simulink model "pioneer_stop_obstacle"  (R2022b)
settings: Solver=ode3  StartTime=0.0  StopTime=inf  FixedStep=0.02  RelTol=1e-3
model workspace (MAT data in the model file):
  Logfile_Data_Object : robotics.ros.BagSelection (value not decoded)
  Logfile_Path = 'C:\Users\user\Desktop\camera2022-04-27-13-31-43.bag'
  Logfile_Playback_Duration = nan
  Logfile_Playback_Offset = nan
undefined symbols (not defined in the file): Angular, Linear, waypoints211
libraries: robotlib x5, robotcorelib x1, robotalgslib x1
settings Model: SimulationMode=external  Creator=user  LastModifiedBy=tarun
settings SolverCC: AlgebraicLoopSolver=TrustRegion
settings OptimizationCC: EnhancedBackFolding=on  PassReuseOutputArgsAs=Individual arguments  ZeroExternalMemoryAtStartup=off  ZeroInternalMemoryAtStartup=off  MaxStackSize=64  OptimizeBlockOrder=speed  DifferentSizesBufferReuse=on  OptimizationCustomize=off  EfficientTunableParamExpr=on
settings DebuggingCC: ParameterTunabilityLossMsg=error  UnconnectedInputMsg=warning  UnconnectedOutputMsg=warning  UnconnectedLineMsg=warning  SFMachineParentedDataDiag=warning
settings HardwareCC: ProdBitPerPointer=32  ProdBitPerSizeT=32  ProdBitPerPtrDiffT=32  ProdLargestAtomicFloat=None  ProdIntDivRoundTo=Undefined  ProdEndianess=Unspecified  ProdWordSize=32  ProdHWDeviceType=Generic->Unspecified (assume 32-bit Generic)
settings ModelReferenceCC: EnableRefExpFcnMdlSchedulingChecks=on
settings SFSimCC: MATLABDynamicMemAlloc=off  SimTargetLang=C++
settings RTWCC: Description=Embedded Coder  SystemTargetFile=ert.tlc  HardwareBoard=Robot Operating System (ROS)  TLCOptions="-aInlineSetEventsForThisBaseRateFcn=TLC_FALSE -aSuppressMultiTaskScheduler=TLC_FALSE  -aRateBasedStepFcn=0"  TemplateMakefile=ert_default_tmf  Toolchain=Catkin  TargetLang=C++  DLArmComputeVersion=19.05
settings CodeAppCC: ForceParamTrailComments=on  IgnoreCustomStorageClasses=off  OperatorAnnotations=on  SimulinkDataObjDesc=on  SFDataObjDesc=on  InsertBlockDesc=on
settings ERTTargetCC: ExtMode=on  ExtModeMexArgs='192.168.232.176' 0 17725

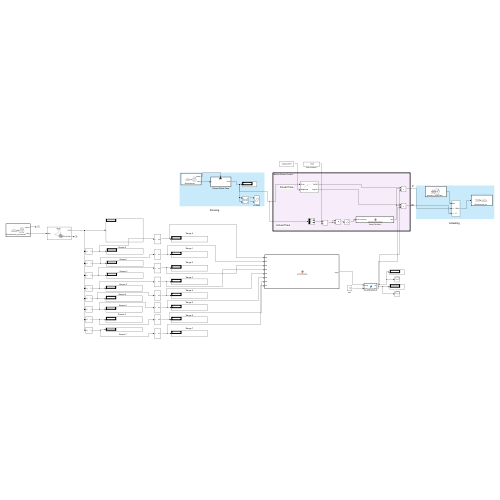
[thumbnail: Simulink's stored preview of the top-level diagram]
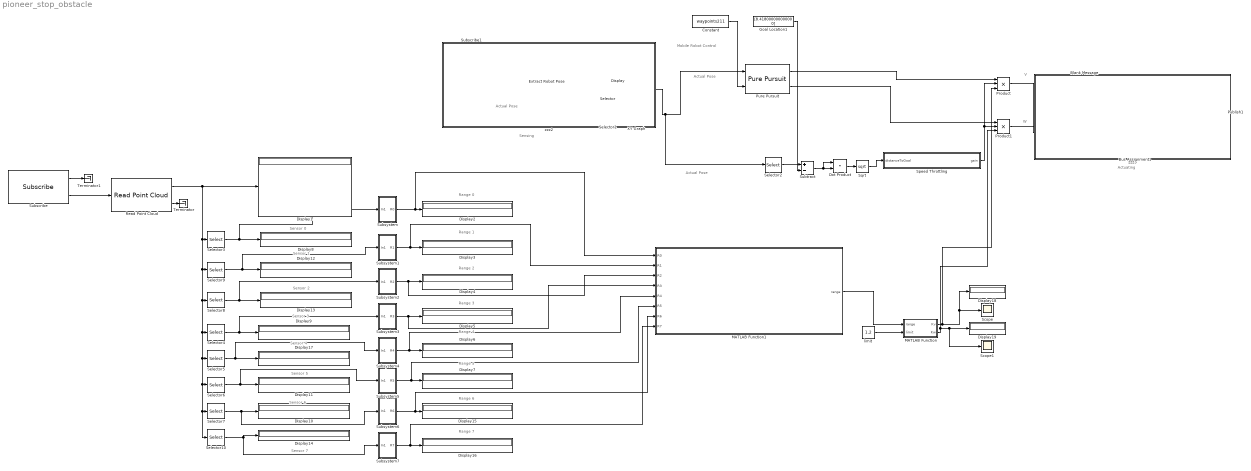
== system pioneer_stop_obstacle ==
  note: Sensing
  note: Sensor 2
  note: Range 6
  note: Actual Pose
  note: Actual Pose
  note: V
  note: Sensor 3
  note: Sensor 4
  note: Mobile Robot Control
  note: Sensor 5
  note: Sensor 0
  note: Range 3
  note: Range 0
  note: Sensor 1
  note: Range 5
  note: Range 7
  note: W
  note: Range 1
  note: Sensor 6
  note: Sensor 7
  note: Range 2
  note: Actual Pose
  note: Range 4
  note: Actuating
  Blank Message : robotlib/Blank Message  messageClass=Message  entityType=geometry_msgs/Twist  messageType=geometry_msgs/Twist  SampleTime=inf  legacyBusStruct=off
  Bus Assignment1 : BusAssignment  AssignedSignals=Linear.X,Angular.Z
  Constant : Constant  Value=waypoints211
  Display{,1..19} (20 alike) : Display
  Dot Product : DotProduct  OutDataTypeStr=Inherit: Inherit via internal rule
  Extract Robot Pose : Subsystem
  Goal Location1 : Constant  Value="[8.41800000000000\t0]"
  MATLAB Function : MATLAB Function  TreatAsAtomicUnit=on
  MATLAB Function1 : MATLAB Function  TreatAsAtomicUnit=on
  Product : Product  Inputs=3
  Product1 : Product  Inputs=3
  Publish1 : robotlib/Publish  topicSource=Select from ROS network  topic=/RosAria/cmd_vel  messageType=geometry_msgs/Twist  legacyBusStruct=off  messageQueueLength=105
  Pure Pursuit : robotalgslib/Pure Pursuit  DesiredLinearVelocity=0.3  MaxAngularVelocity=0.8  LookaheadDistance=1  TargetDirPort=off  SimulateUsing=Code generation
  Read Point Cloud : robotlib/Read Point Cloud  MaximumPointCloudSize=[8, 1]  PreserveStructure=off  ShowRGBOutput=off  ShowIntensityOutput=off  ShowErrorCodeOutput=on  VariableSizeOutputs=off
  Scope : Scope
  Scope1 : Scope
  Selector : Selector  InputPortWidth=3  IndexOptions=Index vector (dialog)  Indices=[1]  OutputSizes=1
  Selector1 : Selector  InputPortWidth=3  IndexOptions=Index vector (dialog)  Indices=[2]  OutputSizes=1
  Selector10 : Selector  NumberOfDimensions=2  InputPortWidth=6  IndexOptions=Starting index (dialog),Starting index (dialog)  Indices=8,1  OutputSizes=1,3
  Selector2 : Selector  InputPortWidth=3  IndexOptions=Index vector (dialog)  Indices=[1 2]  OutputSizes=1
  Selector3 : Selector  NumberOfDimensions=2  InputPortWidth=6  IndexOptions=Starting index (dialog),Starting index (dialog)  Indices=1,1  OutputSizes=1,3
  Selector4 : Selector  NumberOfDimensions=2  InputPortWidth=6  IndexOptions=Starting index (dialog),Starting index (dialog)  Indices=4,1  OutputSizes=1,3
  Selector5 : Selector  NumberOfDimensions=2  InputPortWidth=6  IndexOptions=Starting index (dialog),Starting index (dialog)  Indices=5,1  OutputSizes=1,3
  Selector6 : Selector  NumberOfDimensions=2  InputPortWidth=6  IndexOptions=Starting index (dialog),Starting index (dialog)  Indices=6,1  OutputSizes=1,3
  Selector7 : Selector  NumberOfDimensions=2  InputPortWidth=6  IndexOptions=Starting index (dialog),Starting index (dialog)  Indices=7,1  OutputSizes=1,3
  Selector8 : Selector  NumberOfDimensions=2  InputPortWidth=6  IndexOptions=Starting index (dialog),Starting index (dialog)  Indices=3,1  OutputSizes=1,3
  Selector9 : Selector  NumberOfDimensions=2  InputPortWidth=6  IndexOptions=Starting index (dialog),Starting index (dialog)  Indices=2,1  OutputSizes=1,3
  Speed Throttling : MATLAB Function  TreatAsAtomicUnit=on
  Sqrt : Sqrt
  Subscribe : robotlib/Subscribe  topicSource=Select from ROS network  topic=/RosAria/sonar_pointcloud2  messageType=sensor_msgs/PointCloud2  SampleTime=0.02  legacyBusStruct=off  messageQueueLength=1
  Subscribe1 : robotlib/Subscribe  topicSource=Select from ROS network  topic=/RosAria/pose  messageType=nav_msgs/Odometry  SampleTime=0.02  legacyBusStruct=off  messageQueueLength=51
  Subsystem : Subsystem
  Subsystem1 : Subsystem
  Subsystem2 : Subsystem
  Subsystem3 : Subsystem
  Subsystem4 : Subsystem
  Subsystem5 : Subsystem
  Subsystem6 : Subsystem
  Subsystem7 : Subsystem
  Subtract : Sum  Inputs=+-
  Terminator : Terminator
  Terminator1 : Terminator
  XY Graph : Record  FileSettingsInternal="{\"entries\":[{\"content\":{\"excelSettings\":{\"content\":{},\"type\":\"Streamout.ExcelSettings\"}},\"type\":\"Streamout.FileSettingStorage\",\"uuid\":\"6dcafb8c-c2e8-42d2-a393-42a68d2ab7a7\"}],\"packageUris\":[\"http://schema.mathworks.com/mf0/streamout_blocks/R2020a\"],\"version\":\"1.0\"}"  Layout=[1 1]  SignalsInternal="{\"entries\":[{\"content\":{\"signals\":[{\"content\":{\"blockPath\":[\"pioneer_stop_obstacle/XY Graph\"],\"channel\":[],\"dimensions\":[1],\"domain\":\"pioneer_stop_obstacle/XY Graph\",\"lineColor\":\"#a2142f\",\"plots\":[1],\"port\":1,\"sid\":[],\"signalID\":34,\"signalName\":\"XY Graph:1\"},\"type\":\"RecordBlkView.Signal\",\"uuid\":\"3db1dab7-281e-4972-95fd-2f43a7dd423c\"},{\"content\":{\"blockPath\":[\"pioneer_stop_obstacle/XY Graph\"],\"channel\":[],\"dimensions\":[1],\"domain\":\"pioneer_stop_obstacle/XY Graph\",\"lineColor\":\"#139fff\",\"plots\":[1],\"port\":2,\"sid\":[],\"signalID\":37,\"signalName\":\"XY Graph:2\"},\"type\":\"RecordBlkView.Signal\",\"uuid\":\"8cbd3084-6a6a-4caa-acfe-6605f40577f9\"}]},\"type\":\"RecordBlkView.InputSignals\",\"uuid\":\"3c1224c5-a623-4e21-a2bc-4ee778cdb473\"}],\"packageUris\":[\"http://schema.mathworks.com/mf0/streamout_blocks/R2020a\"],\"version\":\"1.0\"}"  VisualizationBindings="{\"xyplotplugin\":{\"info\":[{\"series\":[{\"bindingParametersList\":[{\"parameter\":\"X-Axis\",\"signalID\":34,\"signalName\":\"XY Graph:1\"},{\"parameter\":\"Y-Axis\",\"signalID\":37,\"signalName\":\"XY Graph:2\"}],\"seriesID\":47604}],\"subplotID\":1}]}}"  CompatibilityTag=XY  st=-1
  limit : Constant  Value=1.2
  zzz2 : Subsystem  TreatAsAtomicUnit=on
      settings: OpenFcn=% no-op
      mask Display: disp('')
  zzz3 : Subsystem  TreatAsAtomicUnit=on
      settings: OpenFcn=% no-op
      mask Display: disp('')
  wires:
  Selector9/1 -> Subsystem1/1(In1), Display12/1
  Subsystem5/1(R5) -> MATLAB Function1/6(R5), Display7/1
  Selector5/1 -> Subsystem4/1(In1), Display17/1
  Selector10/1 -> Subsystem7/1(In1), Display14/1
  Subsystem3/1(R3) -> MATLAB Function1/4(R3), Display5/1
  Selector7/1 -> Subsystem6/1(In1), Display10/1
  Blank Message/1 -> Bus Assignment1/1
  Selector6/1 -> Subsystem5/1(In1), Display11/1
  Subscribe/2 -> Read Point Cloud/1
  Selector/1 -> XY Graph/1
  Read Point Cloud/1 -> Selector10/1, Selector7/1, Selector6/1, Selector5/1, Selector4/1, Selector8/1, Selector9/1, Selector3/1, Display1/1
  Constant/1 -> Pure Pursuit/2
  Product1/1 -> Bus Assignment1/3
  Subsystem7/1(R7) -> MATLAB Function1/8(R7), Display16/1
  Selector3/1 -> Subsystem/1(In1), Display8/1
  Selector4/1 -> Subsystem3/1(In1), Display9/1
  Subsystem6/1(R6) -> MATLAB Function1/7(R6), Display15/1
  Selector1/1 -> XY Graph/2
  Subtract/1 -> Dot Product/1, Dot Product/2
  Product/1 -> Bus Assignment1/2
  Sqrt/1 -> Speed Throttling/1(distanceToGoal)
  Extract Robot Pose/1(Pose) -> Selector/1, Selector1/1, Selector2/1, Pure Pursuit/1, Display/1
  Selector2/1 -> Subtract/1
  Pure Pursuit/2 -> Product1/1
  Subsystem1/1(R1) -> MATLAB Function1/2(R1), Display3/1
  Read Point Cloud/2 -> Terminator/1
  Goal Location1/1 -> Subtract/2
  Speed Throttling/1(gain) -> Product1/2, Product/2
  Pure Pursuit/1 -> Product/1
  Subsystem/1(R0) -> MATLAB Function1/1(R0), Display2/1
  Selector8/1 -> Subsystem2/1(In1), Display13/1
  Subscribe1/1 -> Extract Robot Pose/Enable
  Bus Assignment1/1 -> Publish1/1
  Subsystem2/1(R2) -> MATLAB Function1/3(R2), Display4/1
  Subsystem4/1(R4) -> MATLAB Function1/5(R4), Display6/1
  Subscribe1/2 -> Extract Robot Pose/1(In1)
  Dot Product/1 -> Sqrt/1
  MATLAB Function/1(Kv) -> Product/3, Scope/1, Display18/1
  limit/1 -> MATLAB Function/2(limit)
  MATLAB Function1/1(range) -> MATLAB Function/1(range)
  Subscribe/1 -> Terminator1/1
  MATLAB Function/2(Kw) -> Scope1/1, Display19/1, Product1/3

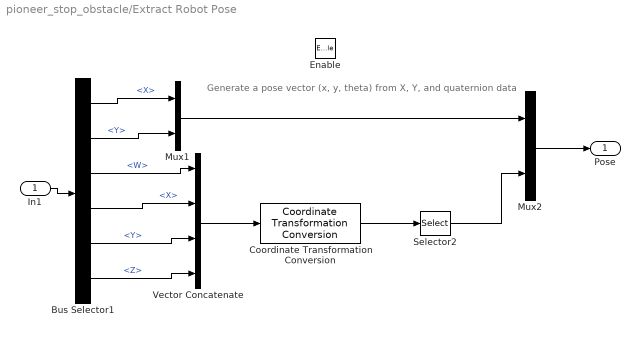
== system pioneer_stop_obstacle/Extract Robot Pose ==
  note: Generate a pose vector (x, y, theta) from X, Y, and quaternion data
  In1 : Inport
  Enable : EnablePort
  Bus Selector1 : BusSelector  OutputSignals=Pose.Pose.Position.X,Pose.Pose.Position.Y,Pose.Pose.Orientation.W,Pose.Pose.Orientation.X,Pose.Pose.Orientation.Y,Pose.Pose.Orientation.Z
  Coordinate Transformation Conversion : robotcorelib/Coordinate Transformation Conversion  InputRepresentation=Quaternion  InputEulerSequence=ZYX  ShowTrVecInputPort=on  OutputRepresentation=Euler Angles  OutputEulerSequence=ZYX  ShowTrVecOutputPort=on  SimulateUsing=Interpreted execution
  Mux1 : Mux  Inputs=2
  Mux2 : Mux  Inputs=2
  Selector2 : Selector  InputPortWidth=3  IndexOptions=Index vector (dialog)  Indices=1  OutputSizes=1
  Vector Concatenate : Concatenate  NumInputs=4
  Pose : Outport  VectorParamsAs1DForOutWhenUnconnected=off
  wires:
  Vector Concatenate/1 -> Coordinate Transformation Conversion/1
  Coordinate Transformation Conversion/1 -> Selector2/1
  Mux1/1 -> Mux2/1
  Selector2/1 -> Mux2/2
  Mux2/1 -> Pose/1
  Bus Selector1/6 -> Vector Concatenate/4  "<Z>"
  Bus Selector1/1 -> Mux1/1  "<X>"
  Bus Selector1/4 -> Vector Concatenate/2  "<X>"
  Bus Selector1/2 -> Mux1/2  "<Y>"
  Bus Selector1/5 -> Vector Concatenate/3  "<Y>"
  In1/1 -> Bus Selector1/1
  Bus Selector1/3 -> Vector Concatenate/1  "<W>"

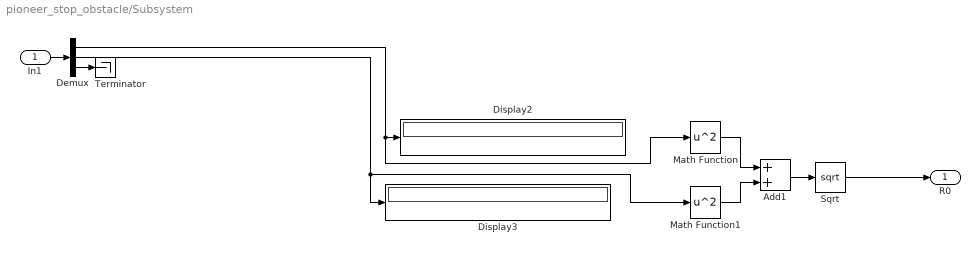
== system pioneer_stop_obstacle/Subsystem ==
  In1 : Inport
  Add1 : Sum
  Demux : Demux  Outputs=3
  Display2 : Display
  Display3 : Display
  Math Function : Math  Operator=square
  Math Function1 : Math  Operator=square
  Sqrt : Sqrt
  Terminator : Terminator
  R0 : Outport
  wires:
  Math Function1/1 -> Add1/2
  Demux/1 -> Math Function/1, Display2/1
  In1/1 -> Demux/1
  Math Function/1 -> Add1/1
  Demux/2 -> Display3/1, Math Function1/1
  Sqrt/1 -> R0/1
  Add1/1 -> Sqrt/1
  Demux/3 -> Terminator/1

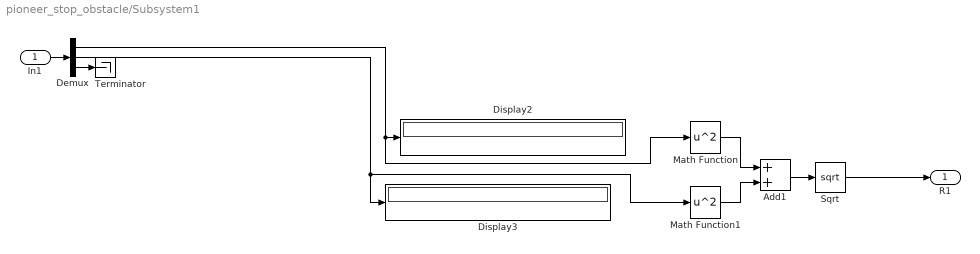
== system pioneer_stop_obstacle/Subsystem1 ==
  In1 : Inport
  Add1 : Sum
  Demux : Demux  Outputs=3
  Display2 : Display
  Display3 : Display
  Math Function : Math  Operator=square
  Math Function1 : Math  Operator=square
  Sqrt : Sqrt
  Terminator : Terminator
  R1 : Outport
  wires:
  Math Function1/1 -> Add1/2
  Demux/1 -> Math Function/1, Display2/1
  In1/1 -> Demux/1
  Math Function/1 -> Add1/1
  Demux/2 -> Display3/1, Math Function1/1
  Sqrt/1 -> R1/1
  Add1/1 -> Sqrt/1
  Demux/3 -> Terminator/1

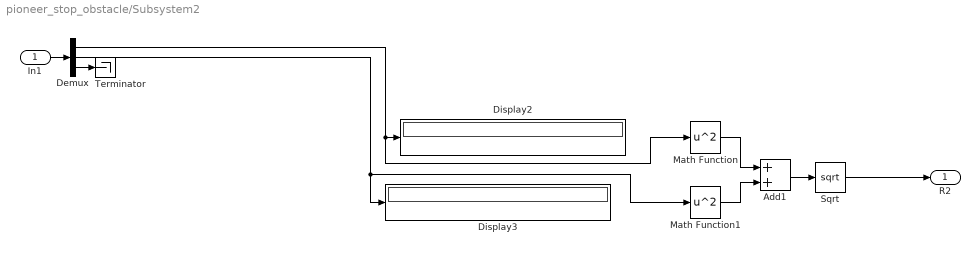
== system pioneer_stop_obstacle/Subsystem2 ==
  In1 : Inport
  Add1 : Sum
  Demux : Demux  Outputs=3
  Display2 : Display
  Display3 : Display
  Math Function : Math  Operator=square
  Math Function1 : Math  Operator=square
  Sqrt : Sqrt
  Terminator : Terminator
  R2 : Outport
  wires:
  Math Function1/1 -> Add1/2
  Demux/1 -> Math Function/1, Display2/1
  In1/1 -> Demux/1
  Math Function/1 -> Add1/1
  Demux/2 -> Display3/1, Math Function1/1
  Sqrt/1 -> R2/1
  Add1/1 -> Sqrt/1
  Demux/3 -> Terminator/1

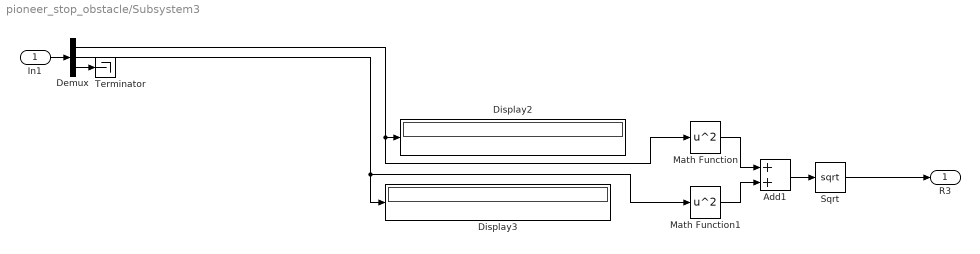
== system pioneer_stop_obstacle/Subsystem3 ==
  In1 : Inport
  Add1 : Sum
  Demux : Demux  Outputs=3
  Display2 : Display
  Display3 : Display
  Math Function : Math  Operator=square
  Math Function1 : Math  Operator=square
  Sqrt : Sqrt
  Terminator : Terminator
  R3 : Outport
  wires:
  Math Function1/1 -> Add1/2
  Demux/1 -> Math Function/1, Display2/1
  In1/1 -> Demux/1
  Math Function/1 -> Add1/1
  Demux/2 -> Display3/1, Math Function1/1
  Sqrt/1 -> R3/1
  Add1/1 -> Sqrt/1
  Demux/3 -> Terminator/1

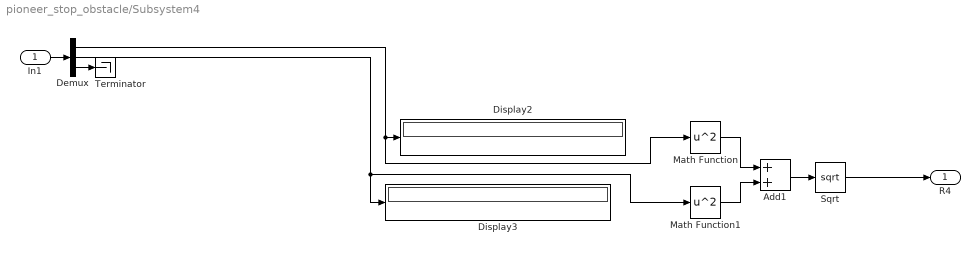
== system pioneer_stop_obstacle/Subsystem4 ==
  In1 : Inport
  Add1 : Sum
  Demux : Demux  Outputs=3
  Display2 : Display
  Display3 : Display
  Math Function : Math  Operator=square
  Math Function1 : Math  Operator=square
  Sqrt : Sqrt
  Terminator : Terminator
  R4 : Outport
  wires:
  Math Function1/1 -> Add1/2
  Demux/1 -> Math Function/1, Display2/1
  In1/1 -> Demux/1
  Math Function/1 -> Add1/1
  Demux/2 -> Display3/1, Math Function1/1
  Sqrt/1 -> R4/1
  Add1/1 -> Sqrt/1
  Demux/3 -> Terminator/1

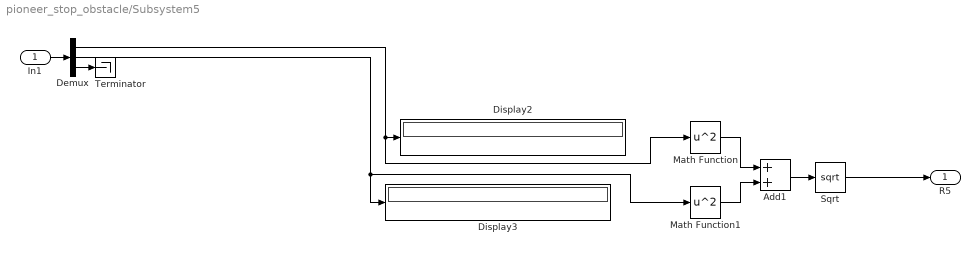
== system pioneer_stop_obstacle/Subsystem5 ==
  In1 : Inport
  Add1 : Sum
  Demux : Demux  Outputs=3
  Display2 : Display
  Display3 : Display
  Math Function : Math  Operator=square
  Math Function1 : Math  Operator=square
  Sqrt : Sqrt
  Terminator : Terminator
  R5 : Outport
  wires:
  Math Function1/1 -> Add1/2
  Demux/1 -> Math Function/1, Display2/1
  In1/1 -> Demux/1
  Math Function/1 -> Add1/1
  Demux/2 -> Display3/1, Math Function1/1
  Sqrt/1 -> R5/1
  Add1/1 -> Sqrt/1
  Demux/3 -> Terminator/1

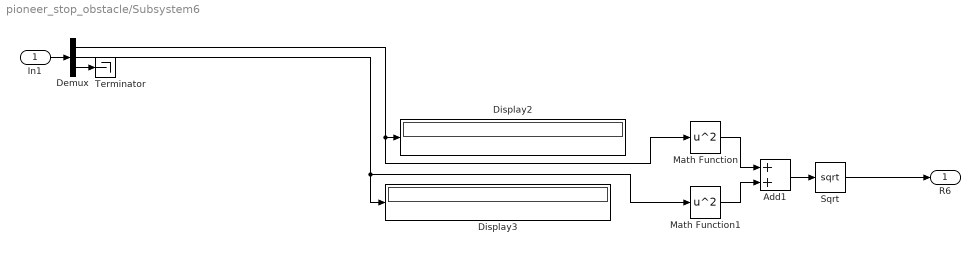
== system pioneer_stop_obstacle/Subsystem6 ==
  In1 : Inport
  Add1 : Sum
  Demux : Demux  Outputs=3
  Display2 : Display
  Display3 : Display
  Math Function : Math  Operator=square
  Math Function1 : Math  Operator=square
  Sqrt : Sqrt
  Terminator : Terminator
  R6 : Outport
  wires:
  Math Function1/1 -> Add1/2
  Demux/1 -> Math Function/1, Display2/1
  In1/1 -> Demux/1
  Math Function/1 -> Add1/1
  Demux/2 -> Display3/1, Math Function1/1
  Sqrt/1 -> R6/1
  Add1/1 -> Sqrt/1
  Demux/3 -> Terminator/1

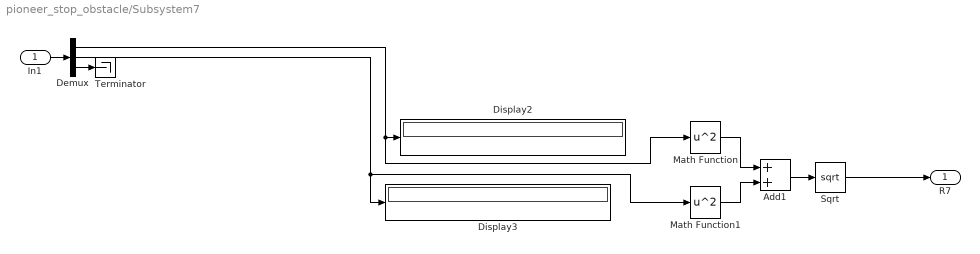
== system pioneer_stop_obstacle/Subsystem7 ==
  In1 : Inport
  Add1 : Sum
  Demux : Demux  Outputs=3
  Display2 : Display
  Display3 : Display
  Math Function : Math  Operator=square
  Math Function1 : Math  Operator=square
  Sqrt : Sqrt
  Terminator : Terminator
  R7 : Outport
  wires:
  Math Function1/1 -> Add1/2
  Demux/1 -> Math Function/1, Display2/1
  In1/1 -> Demux/1
  Math Function/1 -> Add1/1
  Demux/2 -> Display3/1, Math Function1/1
  Sqrt/1 -> R7/1
  Add1/1 -> Sqrt/1
  Demux/3 -> Terminator/1

== system pioneer_stop_obstacle/zzz2 ==

== system pioneer_stop_obstacle/zzz3 ==

== matlab function pioneer_stop_obstacle/Speed Throttling ==
  data: distanceToGoal input; gain output
function gain  = slowDownNearGoal(distanceToGoal)
%%slowDownNearGoal gradually slows the robot when it reaches a goal location.

%continue to move at the normal angular and linear velocity
gain = 1;

%assume that the robot is away from goal
%awayFromGoal = 1;

%threshold to determine if the robot has reached the goal
atGoalThreshold = 0.5;
slowThreshold = 1;

%if the robot is within range and should start slowing down
if(distanceToGoal < slowThreshold)
    
    %speed reduction gain
    gain = distanceToGoal / slowThreshold;
    if(distanceToGoal < atGoalThreshold)
        %stop the robot entirely
        gain = 0;
        %the robot has reached the goal
        %awayFromGoal = 0;
    end
end

== matlab function pioneer_stop_obstacle/MATLAB Function ==
  data: range input; Kv output; limit input; Kw output
 %function [kv,kw] = stopRobot(range,limit)
 %kv=nan;% for the case if the both conditions are false
 %kw=nan;
 %L=limit; %=0.8;% Limit for obstacle
 %t=0;
 %while t=<32
  %   k=(range(4)<L)||(range(5)<L)||(range(6)<L);
  %      if k==false  
  %           kv=1;
  %           kw=1;
  %       else 
  %           kv=0;
  %           kw=0;         
  %       end
  %       t=t+1;
 %end
 


function [Kv,Kw] = stopRobot(range, limit)
%%stopRobot stops the robot based on the sonar sensor. 
Kv = true;
Kw = true;
if range(4)<limit || range(5)<limit || range(6)<limit
    Kv=false;
    Kw=false;
end
%end

== matlab function pioneer_stop_obstacle/MATLAB Function1 ==
  data: R0 input; range output; R1 input; R2 input; R3 input; R4 input; R5 input; R6 input; R7 input
function range = sonarRanges(R0,R1,R2,R3,R4,R5,R6,R7)
range = [R0 R1 R2 R3 R4 R5 R6 R7];
end
